simulink model "Designation"  (R2025b)
settings: Solver=VariableStepAuto  StartTime=0.0  StopTime=Tf  RelTol=1e-3
values from neighbouring files (symbols this model uses):
  Kd = (2*zeta*Wn - Pm) / (Km * Pm)    [Designation_matlab.m]
  Km = 1301    [Designation_matlab.m]
  Kp = Wn^2 / (Km * Pm)    (= 0.106517797472)    [Designation_matlab.m]
  Pm = 10.42    [Designation_matlab.m]
  Ts = 0.005    [Designation_matlab.m]
libraries: simulink x1
settings Model: Creator=ohyus  LastModifiedBy=GILBERT

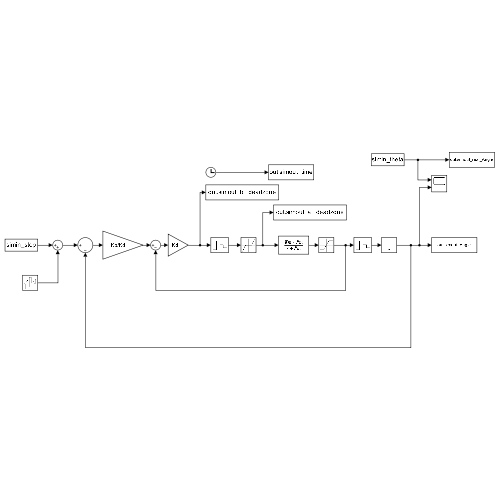
[thumbnail: Simulink's stored preview of the top-level diagram]
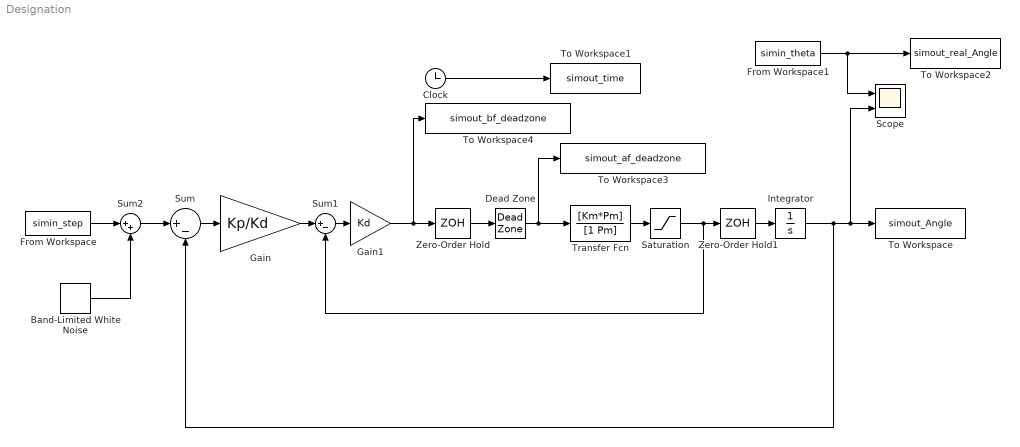
== system Designation ==
  Band-Limited White Noise : simulink/Sources/Band-Limited White Noise  Cov=4*Ts  Ts=Ts  seed=[23341]
  Clock : Clock
  Dead Zone : DeadZone  LowerValue=-0.02  UpperValue=0.02
  From Workspace : FromWorkspace  VariableName=simin_step
  From Workspace1 : FromWorkspace  VariableName=simin_theta
  Gain : Gain  Gain=Kp/Kd
  Gain1 : Gain  Gain=Kd
  Integrator : Integrator
  Saturation : Saturate  UpperLimit=1200  LowerLimit=-1200
  Scope : Scope  NumInputPorts=2
      settings: ActiveDisplayYMinimum=-2.0925382234282459  ActiveDisplayYMaximum=95.620019935803825
  Sum : Sum  Inputs=|+-
  Sum1 : Sum  Inputs=|+-
  Sum2 : Sum  Inputs=|++
  To Workspace : ToWorkspace  VariableName=simout_Angle  SampleTime=-1
  To Workspace1 : ToWorkspace  VariableName=simout_time  SampleTime=-1
  To Workspace2 : ToWorkspace  VariableName=simout_real_Angle  SampleTime=-1
  To Workspace3 : ToWorkspace  VariableName=simout_af_deadzone  SaveFormat=Timeseries  SampleTime=-1
  To Workspace4 : ToWorkspace  VariableName=simout_bf_deadzone  SaveFormat=Timeseries  SampleTime=-1
  Transfer Fcn : TransferFcn  Numerator=[Km*Pm]  Denominator=[1 Pm]
  Zero-Order Hold : ZeroOrderHold  SampleTime=0.005
  Zero-Order Hold1 : ZeroOrderHold  SampleTime=0.005
  wires:
  Sum1/1 -> Gain1/1
  Sum/1 -> Gain/1
  Integrator/1 -> Sum/2, Scope/2, To Workspace/1
  Saturation/1 -> Zero-Order Hold1/1, Sum1/2
  Gain/1 -> Sum1/1
  Transfer Fcn/1 -> Saturation/1
  Gain1/1 -> Zero-Order Hold/1, To Workspace4/1
  Dead Zone/1 -> To Workspace3/1, Transfer Fcn/1
  Clock/1 -> To Workspace1/1
  Band-Limited White Noise/1 -> Sum2/2
  From Workspace/1 -> Sum2/1
  Sum2/1 -> Sum/1
  From Workspace1/1 -> To Workspace2/1, Scope/1
  Zero-Order Hold/1 -> Dead Zone/1
  Zero-Order Hold1/1 -> Integrator/1
